simulink model "half_band"  (Simulink 7.4)
settings: Solver=ode45  StartTime=0.0  StopTime=10.0  RelTol=1e-3
libraries: xbsIndex_r4 x300, casper_library_downconverter x96, casper_library_misc x24
(part 3 of 6)

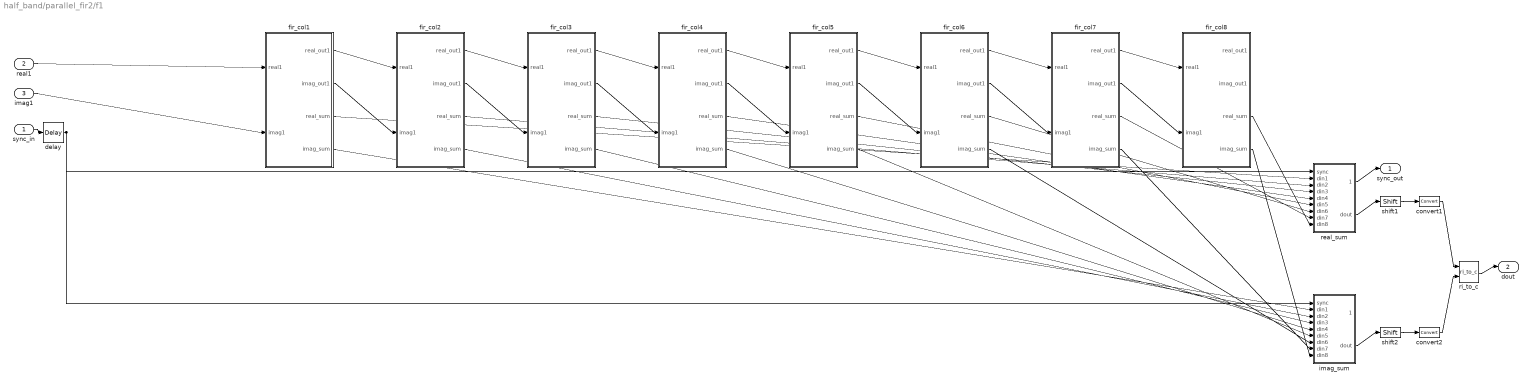
== system half_band/parallel_fir2/f1 ==
  sync_in : Inport
  real1 : Inport  Port=2
  imag1 : Inport  Port=3
  convert1 : xbsIndex_r4/Convert  arith_type="Signed  (2's comp)"  n_bits=4  bin_pt=3  quantization=Truncate  overflow=Wrap  latency=1  dbl_ovrd=off  pipeline=off  block_type=convert
      settings: block_version=10.1.3
  convert2 : xbsIndex_r4/Convert  arith_type="Signed  (2's comp)"  n_bits=4  bin_pt=3  quantization=Truncate  overflow=Wrap  latency=1  dbl_ovrd=off  pipeline=off  block_type=convert
      settings: block_version=10.1.3
  delay : xbsIndex_r4/Delay  en=off  latency=3  dbl_ovrd=off  reg_retiming=off  block_type=delay
  fir_col1 : Subsystem  AncestorBlock=casper_library_downconverter/fir_col  mask(fir_col){n_inputs=1, coeff=0.10000000000000000555111512312578, add_latency=1, mult_latency=2, coeff_bit_width=25, coeff_bin_pt=24, adder_tree_hdl=on}
      mask prompts: n_inputs "Inputs"; coeff "Coefficients"; add_latency "Add latency"; mult_latency "Mult Latency"; coeff_bit_width "Coefficient bit width"; coeff_bin_pt "Coefficient binary point"; adder_tree_hdl "Implement first stage of adder trees on output as behavioural HDL"
      mask init: same as half_band/parallel_fir1/f0/fir_col1
      mask Help: eval('xlWeb(''http://casper.berkeley.edu/wiki/Fir_col'')')
  fir_col2 : Subsystem  AncestorBlock=casper_library_downconverter/fir_col  mask(fir_col){n_inputs=1, coeff=0.20000000000000001110223024625157, add_latency=1, mult_latency=2, coeff_bit_width=25, coeff_bin_pt=24, adder_tree_hdl=on}
      mask prompts: n_inputs "Inputs"; coeff "Coefficients"; add_latency "Add latency"; mult_latency "Mult Latency"; coeff_bit_width "Coefficient bit width"; coeff_bin_pt "Coefficient binary point"; adder_tree_hdl "Implement first stage of adder trees on output as behavioural HDL"
      mask init: same as half_band/parallel_fir1/f0/fir_col1
      mask Help: eval('xlWeb(''http://casper.berkeley.edu/wiki/Fir_col'')')
  fir_col3 : Subsystem  AncestorBlock=casper_library_downconverter/fir_col  mask(fir_col){n_inputs=1, coeff=0.29999999999999998889776975374843, add_latency=1, mult_latency=2, coeff_bit_width=25, coeff_bin_pt=24, adder_tree_hdl=on}
      mask prompts: n_inputs "Inputs"; coeff "Coefficients"; add_latency "Add latency"; mult_latency "Mult Latency"; coeff_bit_width "Coefficient bit width"; coeff_bin_pt "Coefficient binary point"; adder_tree_hdl "Implement first stage of adder trees on output as behavioural HDL"
      mask init: same as half_band/parallel_fir1/f0/fir_col1
      mask Help: eval('xlWeb(''http://casper.berkeley.edu/wiki/Fir_col'')')
  fir_col4 : Subsystem  AncestorBlock=casper_library_downconverter/fir_col  mask(fir_col){n_inputs=1, coeff=0.40000000000000002220446049250313, add_latency=1, mult_latency=2, coeff_bit_width=25, coeff_bin_pt=24, adder_tree_hdl=on}
      mask prompts: n_inputs "Inputs"; coeff "Coefficients"; add_latency "Add latency"; mult_latency "Mult Latency"; coeff_bit_width "Coefficient bit width"; coeff_bin_pt "Coefficient binary point"; adder_tree_hdl "Implement first stage of adder trees on output as behavioural HDL"
      mask init: same as half_band/parallel_fir1/f0/fir_col1
      mask Help: eval('xlWeb(''http://casper.berkeley.edu/wiki/Fir_col'')')
  fir_col5 : Subsystem  AncestorBlock=casper_library_downconverter/fir_col  mask(fir_col){n_inputs=1, coeff=0.5, add_latency=1, mult_latency=2, coeff_bit_width=25, coeff_bin_pt=24, adder_tree_hdl=on}
      mask prompts: n_inputs "Inputs"; coeff "Coefficients"; add_latency "Add latency"; mult_latency "Mult Latency"; coeff_bit_width "Coefficient bit width"; coeff_bin_pt "Coefficient binary point"; adder_tree_hdl "Implement first stage of adder trees on output as behavioural HDL"
      mask init: same as half_band/parallel_fir1/f0/fir_col1
      mask Help: eval('xlWeb(''http://casper.berkeley.edu/wiki/Fir_col'')')
  fir_col6 : Subsystem  AncestorBlock=casper_library_downconverter/fir_col  mask(fir_col){n_inputs=1, coeff=0.59999999999999997779553950749687, add_latency=1, mult_latency=2, coeff_bit_width=25, coeff_bin_pt=24, adder_tree_hdl=on}
      mask prompts: n_inputs "Inputs"; coeff "Coefficients"; add_latency "Add latency"; mult_latency "Mult Latency"; coeff_bit_width "Coefficient bit width"; coeff_bin_pt "Coefficient binary point"; adder_tree_hdl "Implement first stage of adder trees on output as behavioural HDL"
      mask init: same as half_band/parallel_fir1/f0/fir_col1
      mask Help: eval('xlWeb(''http://casper.berkeley.edu/wiki/Fir_col'')')
  fir_col7 : Subsystem  AncestorBlock=casper_library_downconverter/fir_col  mask(fir_col){n_inputs=1, coeff=0.69999999999999995559107901499374, add_latency=1, mult_latency=2, coeff_bit_width=25, coeff_bin_pt=24, adder_tree_hdl=on}
      mask prompts: n_inputs "Inputs"; coeff "Coefficients"; add_latency "Add latency"; mult_latency "Mult Latency"; coeff_bit_width "Coefficient bit width"; coeff_bin_pt "Coefficient binary point"; adder_tree_hdl "Implement first stage of adder trees on output as behavioural HDL"
      mask init: same as half_band/parallel_fir1/f0/fir_col1
      mask Help: eval('xlWeb(''http://casper.berkeley.edu/wiki/Fir_col'')')
  fir_col8 : Subsystem  AncestorBlock=casper_library_downconverter/fir_col  mask(fir_col){n_inputs=1, coeff=0.80000000000000004440892098500626, add_latency=1, mult_latency=2, coeff_bit_width=25, coeff_bin_pt=24, adder_tree_hdl=on}
      mask prompts: n_inputs "Inputs"; coeff "Coefficients"; add_latency "Add latency"; mult_latency "Mult Latency"; coeff_bit_width "Coefficient bit width"; coeff_bin_pt "Coefficient binary point"; adder_tree_hdl "Implement first stage of adder trees on output as behavioural HDL"
      mask init: same as half_band/parallel_fir1/f0/fir_col1
      mask Help: eval('xlWeb(''http://casper.berkeley.edu/wiki/Fir_col'')')
  imag_sum : Subsystem  AncestorBlock=casper_library_misc/adder_tree  mask(adder_tree){n_inputs=8, latency=1, first_stage_hdl=off, behavioral=off}
      mask prompts: n_inputs "Number of Inputs"; latency "Add Latency"; first_stage_hdl "Use behavioural HDL for first stage of adders"; behavioral "Use behavioral HDL for all adders"
      mask help:
      | Sums all inputs using a tree of adds and delays.
      |
      | Number of inputs: The number of inputs to the block to be summed
      | Add latency: The number of clock cycles to perform one addition (affects timing).
      | Use behavioural HDL for first stage of adders: Causes the first stage of adders to be absorbed into DSP blocks if multipliers precede them (Virtex 5).
      | Use behavioural HDL for all adders: Causes all adders in all stages to be implemented in behavioural HDL (may improve timing).
      mask init:
      | adder_tree_init(gcb, ...
      |     'n_inputs', n_inputs, ...
      |     'latency', latency, ...
      |     'first_stage_hdl', first_stage_hdl, ...
      |     'behavioral', behavioral);
      settings: AttributesFormatString=latency 3
      mask Help: eval('xlWeb(''http://casper.berkeley.edu/wiki/Adder_tree'')')
  real_sum : Subsystem  AncestorBlock=casper_library_misc/adder_tree  mask(adder_tree){n_inputs=8, latency=1, first_stage_hdl=off, behavioral=off}
      mask prompts: n_inputs "Number of Inputs"; latency "Add Latency"; first_stage_hdl "Use behavioural HDL for first stage of adders"; behavioral "Use behavioral HDL for all adders"
      mask help:
      | Sums all inputs using a tree of adds and delays.
      |
      | Number of inputs: The number of inputs to the block to be summed
      | Add latency: The number of clock cycles to perform one addition (affects timing).
      | Use behavioural HDL for first stage of adders: Causes the first stage of adders to be absorbed into DSP blocks if multipliers precede them (Virtex 5).
      | Use behavioural HDL for all adders: Causes all adders in all stages to be implemented in behavioural HDL (may improve timing).
      mask init:
      | adder_tree_init(gcb, ...
      |     'n_inputs', n_inputs, ...
      |     'latency', latency, ...
      |     'first_stage_hdl', first_stage_hdl, ...
      |     'behavioral', behavioral);
      settings: AttributesFormatString=latency 3
      mask Help: eval('xlWeb(''http://casper.berkeley.edu/wiki/Adder_tree'')')
  ri_to_c : casper_library_misc/ri_to_c  SystemSampleTime=-1
  shift1 : xbsIndex_r4/Shift  shift_dir=Left  shift_bits=1  en=off  latency=0  precision=Full  arith_type="Signed  (2's comp)"  n_bits=16  bin_pt=14  quantization=Truncate  overflow=Wrap  dbl_ovrd=off  block_type=shift
      settings: block_version=10.1.3
  shift2 : xbsIndex_r4/Shift  shift_dir=Left  shift_bits=1  en=off  latency=0  precision=Full  arith_type="Signed  (2's comp)"  n_bits=16  bin_pt=14  quantization=Truncate  overflow=Wrap  dbl_ovrd=off  block_type=shift
      settings: block_version=10.1.3
  sync_out : Outport
  dout : Outport  Port=2
  wires:
  real_sum/1(sync_out) -> sync_out/1
  delay/1 -> imag_sum/1(sync), real_sum/1(sync)
  sync_in/1 -> delay/1
  ri_to_c/1 -> dout/1
  convert2/1 -> ri_to_c/2
  convert1/1 -> ri_to_c/1
  shift2/1 -> convert2/1
  shift1/1 -> convert1/1
  imag_sum/2(dout) -> shift2/1
  real_sum/2(dout) -> shift1/1
  fir_col8/4(imag_sum) -> imag_sum/9(din8)
  fir_col8/3(real_sum) -> real_sum/9(din8)
  fir_col7/2(imag_out1) -> fir_col8/2(imag1)
  fir_col7/1(real_out1) -> fir_col8/1(real1)
  fir_col7/4(imag_sum) -> imag_sum/8(din7)
  fir_col7/3(real_sum) -> real_sum/8(din7)
  fir_col6/2(imag_out1) -> fir_col7/2(imag1)
  fir_col6/1(real_out1) -> fir_col7/1(real1)
  fir_col6/4(imag_sum) -> imag_sum/7(din6)
  fir_col6/3(real_sum) -> real_sum/7(din6)
  fir_col5/2(imag_out1) -> fir_col6/2(imag1)
  fir_col5/1(real_out1) -> fir_col6/1(real1)
  fir_col5/4(imag_sum) -> imag_sum/6(din5)
  fir_col5/3(real_sum) -> real_sum/6(din5)
  fir_col4/2(imag_out1) -> fir_col5/2(imag1)
  fir_col4/1(real_out1) -> fir_col5/1(real1)
  fir_col4/4(imag_sum) -> imag_sum/5(din4)
  fir_col4/3(real_sum) -> real_sum/5(din4)
  fir_col3/2(imag_out1) -> fir_col4/2(imag1)
  fir_col3/1(real_out1) -> fir_col4/1(real1)
  fir_col3/4(imag_sum) -> imag_sum/4(din3)
  fir_col3/3(real_sum) -> real_sum/4(din3)
  fir_col2/2(imag_out1) -> fir_col3/2(imag1)
  fir_col2/1(real_out1) -> fir_col3/1(real1)
  fir_col2/4(imag_sum) -> imag_sum/3(din2)
  fir_col2/3(real_sum) -> real_sum/3(din2)
  fir_col1/2(imag_out1) -> fir_col2/2(imag1)
  fir_col1/1(real_out1) -> fir_col2/1(real1)
  fir_col1/4(imag_sum) -> imag_sum/2(din1)
  fir_col1/3(real_sum) -> real_sum/2(din1)
  imag1/1 -> fir_col1/2(imag1)
  real1/1 -> fir_col1/1(real1)

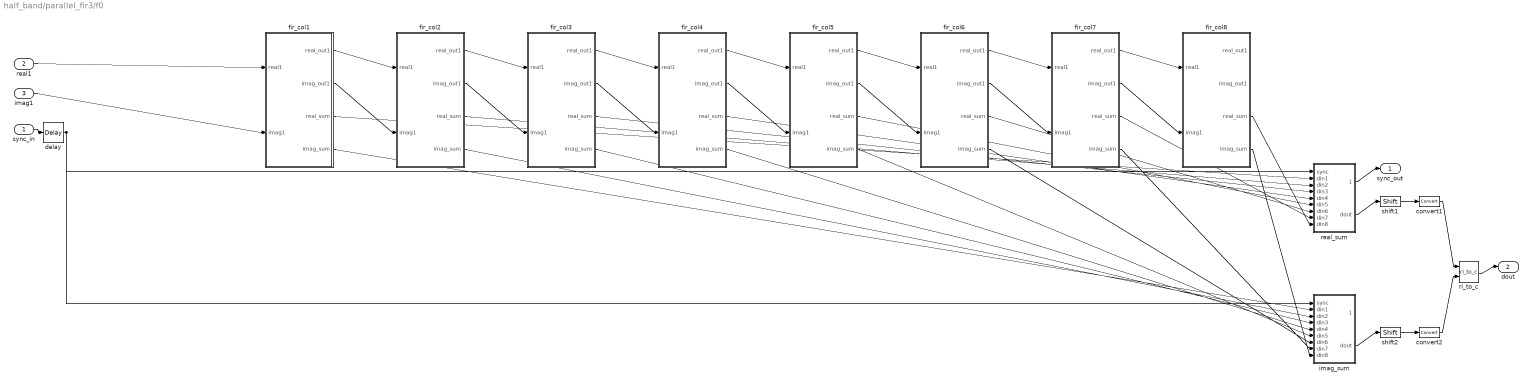
== system half_band/parallel_fir3/f0 ==
  sync_in : Inport
  real1 : Inport  Port=2
  imag1 : Inport  Port=3
  convert1 : xbsIndex_r4/Convert  arith_type="Signed  (2's comp)"  n_bits=4  bin_pt=3  quantization=Truncate  overflow=Wrap  latency=1  dbl_ovrd=off  pipeline=off  block_type=convert
      settings: block_version=10.1.3
  convert2 : xbsIndex_r4/Convert  arith_type="Signed  (2's comp)"  n_bits=4  bin_pt=3  quantization=Truncate  overflow=Wrap  latency=1  dbl_ovrd=off  pipeline=off  block_type=convert
      settings: block_version=10.1.3
  delay : xbsIndex_r4/Delay  en=off  latency=3  dbl_ovrd=off  reg_retiming=off  block_type=delay
  fir_col1 : Subsystem  AncestorBlock=casper_library_downconverter/fir_col  mask(fir_col){n_inputs=1, coeff=0.10000000000000000555111512312578, add_latency=1, mult_latency=2, coeff_bit_width=25, coeff_bin_pt=24, adder_tree_hdl=on}
      mask prompts: n_inputs "Inputs"; coeff "Coefficients"; add_latency "Add latency"; mult_latency "Mult Latency"; coeff_bit_width "Coefficient bit width"; coeff_bin_pt "Coefficient binary point"; adder_tree_hdl "Implement first stage of adder trees on output as behavioural HDL"
      mask init: same as half_band/parallel_fir1/f0/fir_col1
      mask Help: eval('xlWeb(''http://casper.berkeley.edu/wiki/Fir_col'')')
  fir_col2 : Subsystem  AncestorBlock=casper_library_downconverter/fir_col  mask(fir_col){n_inputs=1, coeff=0.20000000000000001110223024625157, add_latency=1, mult_latency=2, coeff_bit_width=25, coeff_bin_pt=24, adder_tree_hdl=on}
      mask prompts: n_inputs "Inputs"; coeff "Coefficients"; add_latency "Add latency"; mult_latency "Mult Latency"; coeff_bit_width "Coefficient bit width"; coeff_bin_pt "Coefficient binary point"; adder_tree_hdl "Implement first stage of adder trees on output as behavioural HDL"
      mask init: same as half_band/parallel_fir1/f0/fir_col1
      mask Help: eval('xlWeb(''http://casper.berkeley.edu/wiki/Fir_col'')')
  fir_col3 : Subsystem  AncestorBlock=casper_library_downconverter/fir_col  mask(fir_col){n_inputs=1, coeff=0.29999999999999998889776975374843, add_latency=1, mult_latency=2, coeff_bit_width=25, coeff_bin_pt=24, adder_tree_hdl=on}
      mask prompts: n_inputs "Inputs"; coeff "Coefficients"; add_latency "Add latency"; mult_latency "Mult Latency"; coeff_bit_width "Coefficient bit width"; coeff_bin_pt "Coefficient binary point"; adder_tree_hdl "Implement first stage of adder trees on output as behavioural HDL"
      mask init: same as half_band/parallel_fir1/f0/fir_col1
      mask Help: eval('xlWeb(''http://casper.berkeley.edu/wiki/Fir_col'')')
  fir_col4 : Subsystem  AncestorBlock=casper_library_downconverter/fir_col  mask(fir_col){n_inputs=1, coeff=0.40000000000000002220446049250313, add_latency=1, mult_latency=2, coeff_bit_width=25, coeff_bin_pt=24, adder_tree_hdl=on}
      mask prompts: n_inputs "Inputs"; coeff "Coefficients"; add_latency "Add latency"; mult_latency "Mult Latency"; coeff_bit_width "Coefficient bit width"; coeff_bin_pt "Coefficient binary point"; adder_tree_hdl "Implement first stage of adder trees on output as behavioural HDL"
      mask init: same as half_band/parallel_fir1/f0/fir_col1
      mask Help: eval('xlWeb(''http://casper.berkeley.edu/wiki/Fir_col'')')
  fir_col5 : Subsystem  AncestorBlock=casper_library_downconverter/fir_col  mask(fir_col){n_inputs=1, coeff=0.5, add_latency=1, mult_latency=2, coeff_bit_width=25, coeff_bin_pt=24, adder_tree_hdl=on}
      mask prompts: n_inputs "Inputs"; coeff "Coefficients"; add_latency "Add latency"; mult_latency "Mult Latency"; coeff_bit_width "Coefficient bit width"; coeff_bin_pt "Coefficient binary point"; adder_tree_hdl "Implement first stage of adder trees on output as behavioural HDL"
      mask init: same as half_band/parallel_fir1/f0/fir_col1
      mask Help: eval('xlWeb(''http://casper.berkeley.edu/wiki/Fir_col'')')
  fir_col6 : Subsystem  AncestorBlock=casper_library_downconverter/fir_col  mask(fir_col){n_inputs=1, coeff=0.59999999999999997779553950749687, add_latency=1, mult_latency=2, coeff_bit_width=25, coeff_bin_pt=24, adder_tree_hdl=on}
      mask prompts: n_inputs "Inputs"; coeff "Coefficients"; add_latency "Add latency"; mult_latency "Mult Latency"; coeff_bit_width "Coefficient bit width"; coeff_bin_pt "Coefficient binary point"; adder_tree_hdl "Implement first stage of adder trees on output as behavioural HDL"
      mask init: same as half_band/parallel_fir1/f0/fir_col1
      mask Help: eval('xlWeb(''http://casper.berkeley.edu/wiki/Fir_col'')')
  fir_col7 : Subsystem  AncestorBlock=casper_library_downconverter/fir_col  mask(fir_col){n_inputs=1, coeff=0.69999999999999995559107901499374, add_latency=1, mult_latency=2, coeff_bit_width=25, coeff_bin_pt=24, adder_tree_hdl=on}
      mask prompts: n_inputs "Inputs"; coeff "Coefficients"; add_latency "Add latency"; mult_latency "Mult Latency"; coeff_bit_width "Coefficient bit width"; coeff_bin_pt "Coefficient binary point"; adder_tree_hdl "Implement first stage of adder trees on output as behavioural HDL"
      mask init: same as half_band/parallel_fir1/f0/fir_col1
      mask Help: eval('xlWeb(''http://casper.berkeley.edu/wiki/Fir_col'')')
  fir_col8 : Subsystem  AncestorBlock=casper_library_downconverter/fir_col  mask(fir_col){n_inputs=1, coeff=0.80000000000000004440892098500626, add_latency=1, mult_latency=2, coeff_bit_width=25, coeff_bin_pt=24, adder_tree_hdl=on}
      mask prompts: n_inputs "Inputs"; coeff "Coefficients"; add_latency "Add latency"; mult_latency "Mult Latency"; coeff_bit_width "Coefficient bit width"; coeff_bin_pt "Coefficient binary point"; adder_tree_hdl "Implement first stage of adder trees on output as behavioural HDL"
      mask init: same as half_band/parallel_fir1/f0/fir_col1
      mask Help: eval('xlWeb(''http://casper.berkeley.edu/wiki/Fir_col'')')
  imag_sum : Subsystem  AncestorBlock=casper_library_misc/adder_tree  mask(adder_tree){n_inputs=8, latency=1, first_stage_hdl=off, behavioral=off}
      mask prompts: n_inputs "Number of Inputs"; latency "Add Latency"; first_stage_hdl "Use behavioural HDL for first stage of adders"; behavioral "Use behavioral HDL for all adders"
      mask help:
      | Sums all inputs using a tree of adds and delays.
      |
      | Number of inputs: The number of inputs to the block to be summed
      | Add latency: The number of clock cycles to perform one addition (affects timing).
      | Use behavioural HDL for first stage of adders: Causes the first stage of adders to be absorbed into DSP blocks if multipliers precede them (Virtex 5).
      | Use behavioural HDL for all adders: Causes all adders in all stages to be implemented in behavioural HDL (may improve timing).
      mask init:
      | adder_tree_init(gcb, ...
      |     'n_inputs', n_inputs, ...
      |     'latency', latency, ...
      |     'first_stage_hdl', first_stage_hdl, ...
      |     'behavioral', behavioral);
      settings: AttributesFormatString=latency 3
      mask Help: eval('xlWeb(''http://casper.berkeley.edu/wiki/Adder_tree'')')
  real_sum : Subsystem  AncestorBlock=casper_library_misc/adder_tree  mask(adder_tree){n_inputs=8, latency=1, first_stage_hdl=off, behavioral=off}
      mask prompts: n_inputs "Number of Inputs"; latency "Add Latency"; first_stage_hdl "Use behavioural HDL for first stage of adders"; behavioral "Use behavioral HDL for all adders"
      mask help:
      | Sums all inputs using a tree of adds and delays.
      |
      | Number of inputs: The number of inputs to the block to be summed
      | Add latency: The number of clock cycles to perform one addition (affects timing).
      | Use behavioural HDL for first stage of adders: Causes the first stage of adders to be absorbed into DSP blocks if multipliers precede them (Virtex 5).
      | Use behavioural HDL for all adders: Causes all adders in all stages to be implemented in behavioural HDL (may improve timing).
      mask init:
      | adder_tree_init(gcb, ...
      |     'n_inputs', n_inputs, ...
      |     'latency', latency, ...
      |     'first_stage_hdl', first_stage_hdl, ...
      |     'behavioral', behavioral);
      settings: AttributesFormatString=latency 3
      mask Help: eval('xlWeb(''http://casper.berkeley.edu/wiki/Adder_tree'')')
  ri_to_c : casper_library_misc/ri_to_c  SystemSampleTime=-1
  shift1 : xbsIndex_r4/Shift  shift_dir=Left  shift_bits=1  en=off  latency=0  precision=Full  arith_type="Signed  (2's comp)"  n_bits=16  bin_pt=14  quantization=Truncate  overflow=Wrap  dbl_ovrd=off  block_type=shift
      settings: block_version=10.1.3
  shift2 : xbsIndex_r4/Shift  shift_dir=Left  shift_bits=1  en=off  latency=0  precision=Full  arith_type="Signed  (2's comp)"  n_bits=16  bin_pt=14  quantization=Truncate  overflow=Wrap  dbl_ovrd=off  block_type=shift
      settings: block_version=10.1.3
  sync_out : Outport
  dout : Outport  Port=2
  wires:
  real_sum/1(sync_out) -> sync_out/1
  delay/1 -> imag_sum/1(sync), real_sum/1(sync)
  sync_in/1 -> delay/1
  ri_to_c/1 -> dout/1
  convert2/1 -> ri_to_c/2
  convert1/1 -> ri_to_c/1
  shift2/1 -> convert2/1
  shift1/1 -> convert1/1
  imag_sum/2(dout) -> shift2/1
  real_sum/2(dout) -> shift1/1
  fir_col8/4(imag_sum) -> imag_sum/9(din8)
  fir_col8/3(real_sum) -> real_sum/9(din8)
  fir_col7/2(imag_out1) -> fir_col8/2(imag1)
  fir_col7/1(real_out1) -> fir_col8/1(real1)
  fir_col7/4(imag_sum) -> imag_sum/8(din7)
  fir_col7/3(real_sum) -> real_sum/8(din7)
  fir_col6/2(imag_out1) -> fir_col7/2(imag1)
  fir_col6/1(real_out1) -> fir_col7/1(real1)
  fir_col6/4(imag_sum) -> imag_sum/7(din6)
  fir_col6/3(real_sum) -> real_sum/7(din6)
  fir_col5/2(imag_out1) -> fir_col6/2(imag1)
  fir_col5/1(real_out1) -> fir_col6/1(real1)
  fir_col5/4(imag_sum) -> imag_sum/6(din5)
  fir_col5/3(real_sum) -> real_sum/6(din5)
  fir_col4/2(imag_out1) -> fir_col5/2(imag1)
  fir_col4/1(real_out1) -> fir_col5/1(real1)
  fir_col4/4(imag_sum) -> imag_sum/5(din4)
  fir_col4/3(real_sum) -> real_sum/5(din4)
  fir_col3/2(imag_out1) -> fir_col4/2(imag1)
  fir_col3/1(real_out1) -> fir_col4/1(real1)
  fir_col3/4(imag_sum) -> imag_sum/4(din3)
  fir_col3/3(real_sum) -> real_sum/4(din3)
  fir_col2/2(imag_out1) -> fir_col3/2(imag1)
  fir_col2/1(real_out1) -> fir_col3/1(real1)
  fir_col2/4(imag_sum) -> imag_sum/3(din2)
  fir_col2/3(real_sum) -> real_sum/3(din2)
  fir_col1/2(imag_out1) -> fir_col2/2(imag1)
  fir_col1/1(real_out1) -> fir_col2/1(real1)
  fir_col1/4(imag_sum) -> imag_sum/2(din1)
  fir_col1/3(real_sum) -> real_sum/2(din1)
  imag1/1 -> fir_col1/2(imag1)
  real1/1 -> fir_col1/1(real1)

== system half_band/parallel_fir3/f0pf1 ==
  sync_in : Inport
  real1 : Inport  Port=2
  imag1 : Inport  Port=3
  convert1 : xbsIndex_r4/Convert  arith_type="Signed  (2's comp)"  n_bits=4  bin_pt=3  quantization=Truncate  overflow=Wrap  latency=1  dbl_ovrd=off  pipeline=off  block_type=convert
      settings: block_version=10.1.3
  convert2 : xbsIndex_r4/Convert  arith_type="Signed  (2's comp)"  n_bits=4  bin_pt=3  quantization=Truncate  overflow=Wrap  latency=1  dbl_ovrd=off  pipeline=off  block_type=convert
      settings: block_version=10.1.3
  delay : xbsIndex_r4/Delay  en=off  latency=3  dbl_ovrd=off  reg_retiming=off  block_type=delay
  fir_col1 : Subsystem  AncestorBlock=casper_library_downconverter/fir_col  mask(fir_col){n_inputs=1, coeff=0.10000000000000000555111512312578, add_latency=1, mult_latency=2, coeff_bit_width=25, coeff_bin_pt=24, adder_tree_hdl=on}
      mask prompts: n_inputs "Inputs"; coeff "Coefficients"; add_latency "Add latency"; mult_latency "Mult Latency"; coeff_bit_width "Coefficient bit width"; coeff_bin_pt "Coefficient binary point"; adder_tree_hdl "Implement first stage of adder trees on output as behavioural HDL"
      mask init: same as half_band/parallel_fir1/f0/fir_col1
      mask Help: eval('xlWeb(''http://casper.berkeley.edu/wiki/Fir_col'')')
  fir_col2 : Subsystem  AncestorBlock=casper_library_downconverter/fir_col  mask(fir_col){n_inputs=1, coeff=0.20000000000000001110223024625157, add_latency=1, mult_latency=2, coeff_bit_width=25, coeff_bin_pt=24, adder_tree_hdl=on}
      mask prompts: n_inputs "Inputs"; coeff "Coefficients"; add_latency "Add latency"; mult_latency "Mult Latency"; coeff_bit_width "Coefficient bit width"; coeff_bin_pt "Coefficient binary point"; adder_tree_hdl "Implement first stage of adder trees on output as behavioural HDL"
      mask init: same as half_band/parallel_fir1/f0/fir_col1
      mask Help: eval('xlWeb(''http://casper.berkeley.edu/wiki/Fir_col'')')
  fir_col3 : Subsystem  AncestorBlock=casper_library_downconverter/fir_col  mask(fir_col){n_inputs=1, coeff=0.29999999999999998889776975374843, add_latency=1, mult_latency=2, coeff_bit_width=25, coeff_bin_pt=24, adder_tree_hdl=on}
      mask prompts: n_inputs "Inputs"; coeff "Coefficients"; add_latency "Add latency"; mult_latency "Mult Latency"; coeff_bit_width "Coefficient bit width"; coeff_bin_pt "Coefficient binary point"; adder_tree_hdl "Implement first stage of adder trees on output as behavioural HDL"
      mask init: same as half_band/parallel_fir1/f0/fir_col1
      mask Help: eval('xlWeb(''http://casper.berkeley.edu/wiki/Fir_col'')')
  fir_col4 : Subsystem  AncestorBlock=casper_library_downconverter/fir_col  mask(fir_col){n_inputs=1, coeff=0.40000000000000002220446049250313, add_latency=1, mult_latency=2, coeff_bit_width=25, coeff_bin_pt=24, adder_tree_hdl=on}
      mask prompts: n_inputs "Inputs"; coeff "Coefficients"; add_latency "Add latency"; mult_latency "Mult Latency"; coeff_bit_width "Coefficient bit width"; coeff_bin_pt "Coefficient binary point"; adder_tree_hdl "Implement first stage of adder trees on output as behavioural HDL"
      mask init: same as half_band/parallel_fir1/f0/fir_col1
      mask Help: eval('xlWeb(''http://casper.berkeley.edu/wiki/Fir_col'')')
  fir_col5 : Subsystem  AncestorBlock=casper_library_downconverter/fir_col  mask(fir_col){n_inputs=1, coeff=0.5, add_latency=1, mult_latency=2, coeff_bit_width=25, coeff_bin_pt=24, adder_tree_hdl=on}
      mask prompts: n_inputs "Inputs"; coeff "Coefficients"; add_latency "Add latency"; mult_latency "Mult Latency"; coeff_bit_width "Coefficient bit width"; coeff_bin_pt "Coefficient binary point"; adder_tree_hdl "Implement first stage of adder trees on output as behavioural HDL"
      mask init: same as half_band/parallel_fir1/f0/fir_col1
      mask Help: eval('xlWeb(''http://casper.berkeley.edu/wiki/Fir_col'')')
  fir_col6 : Subsystem  AncestorBlock=casper_library_downconverter/fir_col  mask(fir_col){n_inputs=1, coeff=0.59999999999999997779553950749687, add_latency=1, mult_latency=2, coeff_bit_width=25, coeff_bin_pt=24, adder_tree_hdl=on}
      mask prompts: n_inputs "Inputs"; coeff "Coefficients"; add_latency "Add latency"; mult_latency "Mult Latency"; coeff_bit_width "Coefficient bit width"; coeff_bin_pt "Coefficient binary point"; adder_tree_hdl "Implement first stage of adder trees on output as behavioural HDL"
      mask init: same as half_band/parallel_fir1/f0/fir_col1
      mask Help: eval('xlWeb(''http://casper.berkeley.edu/wiki/Fir_col'')')
  fir_col7 : Subsystem  AncestorBlock=casper_library_downconverter/fir_col  mask(fir_col){n_inputs=1, coeff=0.69999999999999995559107901499374, add_latency=1, mult_latency=2, coeff_bit_width=25, coeff_bin_pt=24, adder_tree_hdl=on}
      mask prompts: n_inputs "Inputs"; coeff "Coefficients"; add_latency "Add latency"; mult_latency "Mult Latency"; coeff_bit_width "Coefficient bit width"; coeff_bin_pt "Coefficient binary point"; adder_tree_hdl "Implement first stage of adder trees on output as behavioural HDL"
      mask init: same as half_band/parallel_fir1/f0/fir_col1
      mask Help: eval('xlWeb(''http://casper.berkeley.edu/wiki/Fir_col'')')
  fir_col8 : Subsystem  AncestorBlock=casper_library_downconverter/fir_col  mask(fir_col){n_inputs=1, coeff=0.80000000000000004440892098500626, add_latency=1, mult_latency=2, coeff_bit_width=25, coeff_bin_pt=24, adder_tree_hdl=on}
      mask prompts: n_inputs "Inputs"; coeff "Coefficients"; add_latency "Add latency"; mult_latency "Mult Latency"; coeff_bit_width "Coefficient bit width"; coeff_bin_pt "Coefficient binary point"; adder_tree_hdl "Implement first stage of adder trees on output as behavioural HDL"
      mask init: same as half_band/parallel_fir1/f0/fir_col1
      mask Help: eval('xlWeb(''http://casper.berkeley.edu/wiki/Fir_col'')')
  imag_sum : Subsystem  AncestorBlock=casper_library_misc/adder_tree  mask(adder_tree){n_inputs=8, latency=1, first_stage_hdl=off, behavioral=off}
      mask prompts: n_inputs "Number of Inputs"; latency "Add Latency"; first_stage_hdl "Use behavioural HDL for first stage of adders"; behavioral "Use behavioral HDL for all adders"
      mask help:
      | Sums all inputs using a tree of adds and delays.
      |
      | Number of inputs: The number of inputs to the block to be summed
      | Add latency: The number of clock cycles to perform one addition (affects timing).
      | Use behavioural HDL for first stage of adders: Causes the first stage of adders to be absorbed into DSP blocks if multipliers precede them (Virtex 5).
      | Use behavioural HDL for all adders: Causes all adders in all stages to be implemented in behavioural HDL (may improve timing).
      mask init:
      | adder_tree_init(gcb, ...
      |     'n_inputs', n_inputs, ...
      |     'latency', latency, ...
      |     'first_stage_hdl', first_stage_hdl, ...
      |     'behavioral', behavioral);
      settings: AttributesFormatString=latency 3
      mask Help: eval('xlWeb(''http://casper.berkeley.edu/wiki/Adder_tree'')')
  real_sum : Subsystem  AncestorBlock=casper_library_misc/adder_tree  mask(adder_tree){n_inputs=8, latency=1, first_stage_hdl=off, behavioral=off}
      mask prompts: n_inputs "Number of Inputs"; latency "Add Latency"; first_stage_hdl "Use behavioural HDL for first stage of adders"; behavioral "Use behavioral HDL for all adders"
      mask help:
      | Sums all inputs using a tree of adds and delays.
      |
      | Number of inputs: The number of inputs to the block to be summed
      | Add latency: The number of clock cycles to perform one addition (affects timing).
      | Use behavioural HDL for first stage of adders: Causes the first stage of adders to be absorbed into DSP blocks if multipliers precede them (Virtex 5).
      | Use behavioural HDL for all adders: Causes all adders in all stages to be implemented in behavioural HDL (may improve timing).
      mask init:
      | adder_tree_init(gcb, ...
      |     'n_inputs', n_inputs, ...
      |     'latency', latency, ...
      |     'first_stage_hdl', first_stage_hdl, ...
      |     'behavioral', behavioral);
      settings: AttributesFormatString=latency 3
      mask Help: eval('xlWeb(''http://casper.berkeley.edu/wiki/Adder_tree'')')
  ri_to_c : casper_library_misc/ri_to_c  SystemSampleTime=-1
  shift1 : xbsIndex_r4/Shift  shift_dir=Left  shift_bits=1  en=off  latency=0  precision=Full  arith_type="Signed  (2's comp)"  n_bits=16  bin_pt=14  quantization=Truncate  overflow=Wrap  dbl_ovrd=off  block_type=shift
      settings: block_version=10.1.3
  shift2 : xbsIndex_r4/Shift  shift_dir=Left  shift_bits=1  en=off  latency=0  precision=Full  arith_type="Signed  (2's comp)"  n_bits=16  bin_pt=14  quantization=Truncate  overflow=Wrap  dbl_ovrd=off  block_type=shift
      settings: block_version=10.1.3
  sync_out : Outport
  dout : Outport  Port=2
  wires:
  real1/1 -> fir_col1/1(real1)
  imag1/1 -> fir_col1/2(imag1)
  fir_col1/3(real_sum) -> real_sum/2(din1)
  fir_col1/4(imag_sum) -> imag_sum/2(din1)
  fir_col1/1(real_out1) -> fir_col2/1(real1)
  fir_col1/2(imag_out1) -> fir_col2/2(imag1)
  fir_col2/3(real_sum) -> real_sum/3(din2)
  fir_col2/4(imag_sum) -> imag_sum/3(din2)
  fir_col2/1(real_out1) -> fir_col3/1(real1)
  fir_col2/2(imag_out1) -> fir_col3/2(imag1)
  fir_col3/3(real_sum) -> real_sum/4(din3)
  fir_col3/4(imag_sum) -> imag_sum/4(din3)
  fir_col3/1(real_out1) -> fir_col4/1(real1)
  fir_col3/2(imag_out1) -> fir_col4/2(imag1)
  fir_col4/3(real_sum) -> real_sum/5(din4)
  fir_col4/4(imag_sum) -> imag_sum/5(din4)
  fir_col4/1(real_out1) -> fir_col5/1(real1)
  fir_col4/2(imag_out1) -> fir_col5/2(imag1)
  fir_col5/3(real_sum) -> real_sum/6(din5)
  fir_col5/4(imag_sum) -> imag_sum/6(din5)
  fir_col5/1(real_out1) -> fir_col6/1(real1)
  fir_col5/2(imag_out1) -> fir_col6/2(imag1)
  fir_col6/3(real_sum) -> real_sum/7(din6)
  fir_col6/4(imag_sum) -> imag_sum/7(din6)
  fir_col6/1(real_out1) -> fir_col7/1(real1)
  fir_col6/2(imag_out1) -> fir_col7/2(imag1)
  fir_col7/3(real_sum) -> real_sum/8(din7)
  fir_col7/4(imag_sum) -> imag_sum/8(din7)
  fir_col7/1(real_out1) -> fir_col8/1(real1)
  fir_col7/2(imag_out1) -> fir_col8/2(imag1)
  fir_col8/3(real_sum) -> real_sum/9(din8)
  fir_col8/4(imag_sum) -> imag_sum/9(din8)
  real_sum/2(dout) -> shift1/1
  imag_sum/2(dout) -> shift2/1
  shift1/1 -> convert1/1
  shift2/1 -> convert2/1
  convert1/1 -> ri_to_c/1
  convert2/1 -> ri_to_c/2
  ri_to_c/1 -> dout/1
  sync_in/1 -> delay/1
  delay/1 -> real_sum/1(sync), imag_sum/1(sync)
  real_sum/1(sync_out) -> sync_out/1

== system half_band/parallel_fir3/f1 ==
  sync_in : Inport
  real1 : Inport  Port=2
  imag1 : Inport  Port=3
  convert1 : xbsIndex_r4/Convert  arith_type="Signed  (2's comp)"  n_bits=4  bin_pt=3  quantization=Truncate  overflow=Wrap  latency=1  dbl_ovrd=off  pipeline=off  block_type=convert
      settings: block_version=10.1.3
  convert2 : xbsIndex_r4/Convert  arith_type="Signed  (2's comp)"  n_bits=4  bin_pt=3  quantization=Truncate  overflow=Wrap  latency=1  dbl_ovrd=off  pipeline=off  block_type=convert
      settings: block_version=10.1.3
  delay : xbsIndex_r4/Delay  en=off  latency=3  dbl_ovrd=off  reg_retiming=off  block_type=delay
  fir_col1 : Subsystem  AncestorBlock=casper_library_downconverter/fir_col  mask(fir_col){n_inputs=1, coeff=0.10000000000000000555111512312578, add_latency=1, mult_latency=2, coeff_bit_width=25, coeff_bin_pt=24, adder_tree_hdl=on}
      mask prompts: n_inputs "Inputs"; coeff "Coefficients"; add_latency "Add latency"; mult_latency "Mult Latency"; coeff_bit_width "Coefficient bit width"; coeff_bin_pt "Coefficient binary point"; adder_tree_hdl "Implement first stage of adder trees on output as behavioural HDL"
      mask init: same as half_band/parallel_fir1/f0/fir_col1
      mask Help: eval('xlWeb(''http://casper.berkeley.edu/wiki/Fir_col'')')
  fir_col2 : Subsystem  AncestorBlock=casper_library_downconverter/fir_col  mask(fir_col){n_inputs=1, coeff=0.20000000000000001110223024625157, add_latency=1, mult_latency=2, coeff_bit_width=25, coeff_bin_pt=24, adder_tree_hdl=on}
      mask prompts: n_inputs "Inputs"; coeff "Coefficients"; add_latency "Add latency"; mult_latency "Mult Latency"; coeff_bit_width "Coefficient bit width"; coeff_bin_pt "Coefficient binary point"; adder_tree_hdl "Implement first stage of adder trees on output as behavioural HDL"
      mask init: same as half_band/parallel_fir1/f0/fir_col1
      mask Help: eval('xlWeb(''http://casper.berkeley.edu/wiki/Fir_col'')')
  fir_col3 : Subsystem  AncestorBlock=casper_library_downconverter/fir_col  mask(fir_col){n_inputs=1, coeff=0.29999999999999998889776975374843, add_latency=1, mult_latency=2, coeff_bit_width=25, coeff_bin_pt=24, adder_tree_hdl=on}
      mask prompts: n_inputs "Inputs"; coeff "Coefficients"; add_latency "Add latency"; mult_latency "Mult Latency"; coeff_bit_width "Coefficient bit width"; coeff_bin_pt "Coefficient binary point"; adder_tree_hdl "Implement first stage of adder trees on output as behavioural HDL"
      mask init: same as half_band/parallel_fir1/f0/fir_col1
      mask Help: eval('xlWeb(''http://casper.berkeley.edu/wiki/Fir_col'')')
  fir_col4 : Subsystem  AncestorBlock=casper_library_downconverter/fir_col  mask(fir_col){n_inputs=1, coeff=0.40000000000000002220446049250313, add_latency=1, mult_latency=2, coeff_bit_width=25, coeff_bin_pt=24, adder_tree_hdl=on}
      mask prompts: n_inputs "Inputs"; coeff "Coefficients"; add_latency "Add latency"; mult_latency "Mult Latency"; coeff_bit_width "Coefficient bit width"; coeff_bin_pt "Coefficient binary point"; adder_tree_hdl "Implement first stage of adder trees on output as behavioural HDL"
      mask init: same as half_band/parallel_fir1/f0/fir_col1
      mask Help: eval('xlWeb(''http://casper.berkeley.edu/wiki/Fir_col'')')
  fir_col5 : Subsystem  AncestorBlock=casper_library_downconverter/fir_col  mask(fir_col){n_inputs=1, coeff=0.5, add_latency=1, mult_latency=2, coeff_bit_width=25, coeff_bin_pt=24, adder_tree_hdl=on}
      mask prompts: n_inputs "Inputs"; coeff "Coefficients"; add_latency "Add latency"; mult_latency "Mult Latency"; coeff_bit_width "Coefficient bit width"; coeff_bin_pt "Coefficient binary point"; adder_tree_hdl "Implement first stage of adder trees on output as behavioural HDL"
      mask init: same as half_band/parallel_fir1/f0/fir_col1
      mask Help: eval('xlWeb(''http://casper.berkeley.edu/wiki/Fir_col'')')
  fir_col6 : Subsystem  AncestorBlock=casper_library_downconverter/fir_col  mask(fir_col){n_inputs=1, coeff=0.59999999999999997779553950749687, add_latency=1, mult_latency=2, coeff_bit_width=25, coeff_bin_pt=24, adder_tree_hdl=on}
      mask prompts: n_inputs "Inputs"; coeff "Coefficients"; add_latency "Add latency"; mult_latency "Mult Latency"; coeff_bit_width "Coefficient bit width"; coeff_bin_pt "Coefficient binary point"; adder_tree_hdl "Implement first stage of adder trees on output as behavioural HDL"
      mask init: same as half_band/parallel_fir1/f0/fir_col1
      mask Help: eval('xlWeb(''http://casper.berkeley.edu/wiki/Fir_col'')')
  fir_col7 : Subsystem  AncestorBlock=casper_library_downconverter/fir_col  mask(fir_col){n_inputs=1, coeff=0.69999999999999995559107901499374, add_latency=1, mult_latency=2, coeff_bit_width=25, coeff_bin_pt=24, adder_tree_hdl=on}
      mask prompts: n_inputs "Inputs"; coeff "Coefficients"; add_latency "Add latency"; mult_latency "Mult Latency"; coeff_bit_width "Coefficient bit width"; coeff_bin_pt "Coefficient binary point"; adder_tree_hdl "Implement first stage of adder trees on output as behavioural HDL"
      mask init: same as half_band/parallel_fir1/f0/fir_col1
      mask Help: eval('xlWeb(''http://casper.berkeley.edu/wiki/Fir_col'')')
  fir_col8 : Subsystem  AncestorBlock=casper_library_downconverter/fir_col  mask(fir_col){n_inputs=1, coeff=0.80000000000000004440892098500626, add_latency=1, mult_latency=2, coeff_bit_width=25, coeff_bin_pt=24, adder_tree_hdl=on}
      mask prompts: n_inputs "Inputs"; coeff "Coefficients"; add_latency "Add latency"; mult_latency "Mult Latency"; coeff_bit_width "Coefficient bit width"; coeff_bin_pt "Coefficient binary point"; adder_tree_hdl "Implement first stage of adder trees on output as behavioural HDL"
      mask init: same as half_band/parallel_fir1/f0/fir_col1
      mask Help: eval('xlWeb(''http://casper.berkeley.edu/wiki/Fir_col'')')
  imag_sum : Subsystem  AncestorBlock=casper_library_misc/adder_tree  mask(adder_tree){n_inputs=8, latency=1, first_stage_hdl=off, behavioral=off}
      mask prompts: n_inputs "Number of Inputs"; latency "Add Latency"; first_stage_hdl "Use behavioural HDL for first stage of adders"; behavioral "Use behavioral HDL for all adders"
      mask help:
      | Sums all inputs using a tree of adds and delays.
      |
      | Number of inputs: The number of inputs to the block to be summed
      | Add latency: The number of clock cycles to perform one addition (affects timing).
      | Use behavioural HDL for first stage of adders: Causes the first stage of adders to be absorbed into DSP blocks if multipliers precede them (Virtex 5).
      | Use behavioural HDL for all adders: Causes all adders in all stages to be implemented in behavioural HDL (may improve timing).
      mask init:
      | adder_tree_init(gcb, ...
      |     'n_inputs', n_inputs, ...
      |     'latency', latency, ...
      |     'first_stage_hdl', first_stage_hdl, ...
      |     'behavioral', behavioral);
      settings: AttributesFormatString=latency 3
      mask Help: eval('xlWeb(''http://casper.berkeley.edu/wiki/Adder_tree'')')
  real_sum : Subsystem  AncestorBlock=casper_library_misc/adder_tree  mask(adder_tree){n_inputs=8, latency=1, first_stage_hdl=off, behavioral=off}
      mask prompts: n_inputs "Number of Inputs"; latency "Add Latency"; first_stage_hdl "Use behavioural HDL for first stage of adders"; behavioral "Use behavioral HDL for all adders"
      mask help:
      | Sums all inputs using a tree of adds and delays.
      |
      | Number of inputs: The number of inputs to the block to be summed
      | Add latency: The number of clock cycles to perform one addition (affects timing).
      | Use behavioural HDL for first stage of adders: Causes the first stage of adders to be absorbed into DSP blocks if multipliers precede them (Virtex 5).
      | Use behavioural HDL for all adders: Causes all adders in all stages to be implemented in behavioural HDL (may improve timing).
      mask init:
      | adder_tree_init(gcb, ...
      |     'n_inputs', n_inputs, ...
      |     'latency', latency, ...
      |     'first_stage_hdl', first_stage_hdl, ...
      |     'behavioral', behavioral);
      settings: AttributesFormatString=latency 3
      mask Help: eval('xlWeb(''http://casper.berkeley.edu/wiki/Adder_tree'')')
  ri_to_c : casper_library_misc/ri_to_c  SystemSampleTime=-1
  shift1 : xbsIndex_r4/Shift  shift_dir=Left  shift_bits=1  en=off  latency=0  precision=Full  arith_type="Signed  (2's comp)"  n_bits=16  bin_pt=14  quantization=Truncate  overflow=Wrap  dbl_ovrd=off  block_type=shift
      settings: block_version=10.1.3
  shift2 : xbsIndex_r4/Shift  shift_dir=Left  shift_bits=1  en=off  latency=0  precision=Full  arith_type="Signed  (2's comp)"  n_bits=16  bin_pt=14  quantization=Truncate  overflow=Wrap  dbl_ovrd=off  block_type=shift
      settings: block_version=10.1.3
  sync_out : Outport
  dout : Outport  Port=2
  wires:
  real_sum/1(sync_out) -> sync_out/1
  delay/1 -> imag_sum/1(sync), real_sum/1(sync)
  sync_in/1 -> delay/1
  ri_to_c/1 -> dout/1
  convert2/1 -> ri_to_c/2
  convert1/1 -> ri_to_c/1
  shift2/1 -> convert2/1
  shift1/1 -> convert1/1
  imag_sum/2(dout) -> shift2/1
  real_sum/2(dout) -> shift1/1
  fir_col8/4(imag_sum) -> imag_sum/9(din8)
  fir_col8/3(real_sum) -> real_sum/9(din8)
  fir_col7/2(imag_out1) -> fir_col8/2(imag1)
  fir_col7/1(real_out1) -> fir_col8/1(real1)
  fir_col7/4(imag_sum) -> imag_sum/8(din7)
  fir_col7/3(real_sum) -> real_sum/8(din7)
  fir_col6/2(imag_out1) -> fir_col7/2(imag1)
  fir_col6/1(real_out1) -> fir_col7/1(real1)
  fir_col6/4(imag_sum) -> imag_sum/7(din6)
  fir_col6/3(real_sum) -> real_sum/7(din6)
  fir_col5/2(imag_out1) -> fir_col6/2(imag1)
  fir_col5/1(real_out1) -> fir_col6/1(real1)
  fir_col5/4(imag_sum) -> imag_sum/6(din5)
  fir_col5/3(real_sum) -> real_sum/6(din5)
  fir_col4/2(imag_out1) -> fir_col5/2(imag1)
  fir_col4/1(real_out1) -> fir_col5/1(real1)
  fir_col4/4(imag_sum) -> imag_sum/5(din4)
  fir_col4/3(real_sum) -> real_sum/5(din4)
  fir_col3/2(imag_out1) -> fir_col4/2(imag1)
  fir_col3/1(real_out1) -> fir_col4/1(real1)
  fir_col3/4(imag_sum) -> imag_sum/4(din3)
  fir_col3/3(real_sum) -> real_sum/4(din3)
  fir_col2/2(imag_out1) -> fir_col3/2(imag1)
  fir_col2/1(real_out1) -> fir_col3/1(real1)
  fir_col2/4(imag_sum) -> imag_sum/3(din2)
  fir_col2/3(real_sum) -> real_sum/3(din2)
  fir_col1/2(imag_out1) -> fir_col2/2(imag1)
  fir_col1/1(real_out1) -> fir_col2/1(real1)
  fir_col1/4(imag_sum) -> imag_sum/2(din1)
  fir_col1/3(real_sum) -> real_sum/2(din1)
  imag1/1 -> fir_col1/2(imag1)
  real1/1 -> fir_col1/1(real1)
